simulink subsystem "Encoder1D"  (R2024a)
settings: Solver=VariableStepAuto  StartTime=0.0  StopTime=10.0  RelTol=1e-3
undefined symbols (not defined in the file or in its folder): ABPhase, gearReductionRatio, PPR, wheelRadius
settings Model: Creator=Peter  LastModifiedBy=Peter

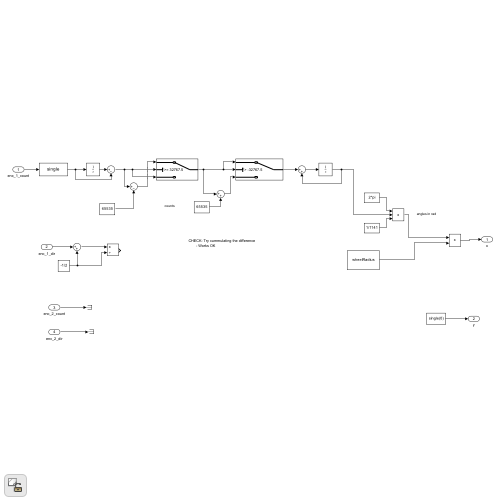
[thumbnail: Simulink's stored preview of the top-level diagram]
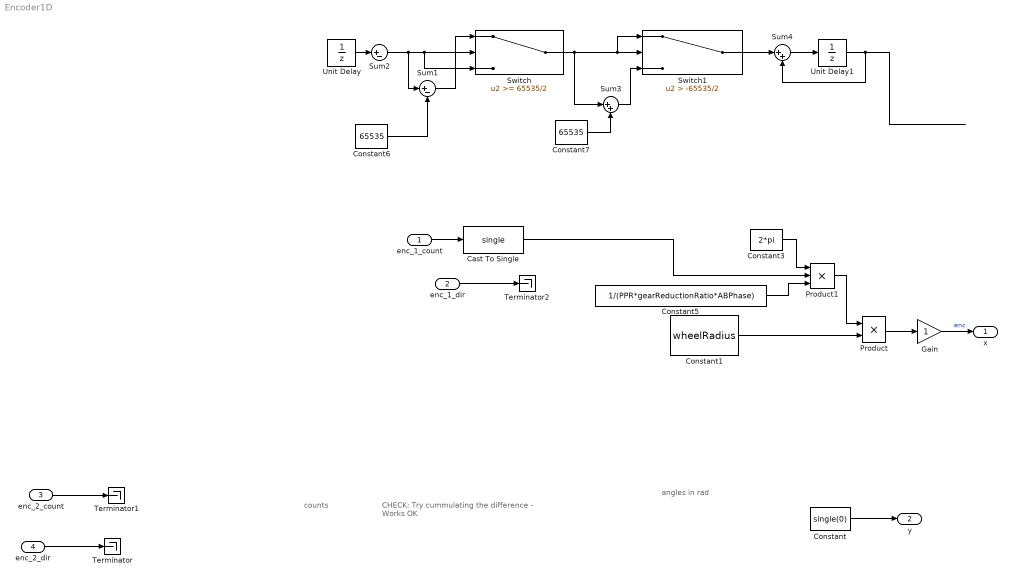
== system Encoder1D ==
  note: CHECK: Try cummulating the difference
      | 	- Works OK
  note: counts
  note: angles in rad
  enc_1_count : Inport
  enc_1_dir : Inport  Port=2
  enc_2_count : Inport  Port=3
  enc_2_dir : Inport  Port=4
  Cast To Single : DataTypeConversion  OutDataTypeStr=single  SaturateOnIntegerOverflow=off  RndMeth=Floor
  Constant : Constant  Value=single(0)  OutDataTypeStr=single
  Constant1 : Constant  Value=wheelRadius
  Constant3 : Constant  Value=2*pi  OutDataTypeStr=single
  Constant5 : Constant  Value=1/(PPR*gearReductionRatio*ABPhase)  OutDataTypeStr=single
  Constant6 : Constant  Value=65535  OutDataTypeStr=single
  Constant7 : Constant  Value=65535  OutDataTypeStr=single
  Gain : Gain
  Product : Product  OutDataTypeStr=single
  Product1 : Product  Inputs=3  OutDataTypeStr=single
  Sum1 : Sum  Inputs=|+-
  Sum2 : Sum  Inputs=|+-  OutDataTypeStr=single  AccumDataTypeStr=single
  Sum3 : Sum  Inputs=|++
  Sum4 : Sum  Inputs=|++
  Switch : Switch  Threshold=65535/2  SaturateOnIntegerOverflow=off  InputSameDT=off
  Switch1 : Switch  Criteria=u2 > Threshold  Threshold=-65535/2  SaturateOnIntegerOverflow=off  InputSameDT=off
  Terminator : Terminator
  Terminator1 : Terminator
  Terminator2 : Terminator
  Unit Delay : UnitDelay  SampleTime=-1  HasFrameUpgradeWarning=on
  Unit Delay1 : UnitDelay  SampleTime=-1  HasFrameUpgradeWarning=on
  x : Outport  OutDataTypeStr=single
  y : Outport  Port=2  OutDataTypeStr=single
  wires:
  enc_2_dir/1 -> Terminator/1
  Constant/1 -> y/1
  Product1/1 -> Product/1
  enc_2_count/1 -> Terminator1/1
  Constant5/1 -> Product1/3
  Constant3/1 -> Product1/1
  Product/1 -> Gain/1
  Constant1/1 -> Product/2
  Cast To Single/1 -> Product1/2
  enc_1_count/1 -> Cast To Single/1
  Gain/1 -> x/1  "enc"
  enc_1_dir/1 -> Terminator2/1
  Sum2/1 -> Switch/2, Switch/3, Sum1/1
  Unit Delay1/1 -> Sum4/2
  Sum4/1 -> Unit Delay1/1
  ? -> Sum2/2
  Unit Delay/1 -> Sum2/1
  Switch1/1 -> Sum4/1
  Switch/1 -> Switch1/2, Switch1/1, Sum3/1
  Sum3/1 -> Switch1/3
  Constant6/1 -> Sum1/2
  Constant7/1 -> Sum3/2
  Sum1/1 -> Switch/1
  ? -> Unit Delay/1
